simulink model "Controller_Pioneer3DXAssembly"  (R2019b)
settings: Solver=ode45  StartTime=0.0  StopTime=200  RelTol=1e-3  EnableMultiTasking=on
InitFcn:
  | load WorldLUTData.mat
  | r = 0.095; %Wheel radius
  | b = 0.33; %Wheel base
undefined symbols (not defined in the file): World_LUT, X, Y, Z
libraries: sm_lib x35, nesl_utility x19, fl_lib x3, fl_ps_legacy_lib x3, vrlib x2
(part 2 of 2)

== system Controller_Pioneer3DXAssembly/Wheel Right/WheelMain_1_RIGID ==
  ReferenceFrame : sm_lib/Frames and Transforms/Reference Frame
  Solid : sm_lib/Body Elements/File Solid  ExtGeomFileName=WheelMain_Default_sldprt.STL  UnitType=FromFile  ExtGeomFileUnits=in  StepReaderType=HEX  ExportEntireGeometry=off  InertiaType=Custom  Mass=0.95054099999999997  MassUnits=kg  CenterOfMass=[6.6644881889763772 2.3641220472440942e-11 0.063999999999999987]  CenterOfMassUnits=in  MomentsOfInertia=[7.7667865335730646 4.0958211916423819 4.0958211916423819]  MomentsOfInertiaUnits=kg*in^2  ProductsOfInertia=[-2.8456041912083817e-11 2.5874201748403487e-11 1.023105896211792e-11]  ProductsOfInertiaUnits=kg*in^2  BasedOnType=Density  Density=1000  DensityUnits=kg/(m^3)  DoExposeReferenceFrame=on  SerializedFrames=<Frames/>  GraphicType=FromGeometry  MarkerShape=Sphere  MarkerSize=10  MarkerSizeUnits=m  GraphicVisPropType=SimpleVisualProperties  GraphicDiffuseColor=[0.792157 0.819608 0.933333]  GraphicSpecularColor=[0.5 0.5 0.5 1.0]  GraphicAmbientColor=[0.15 0.15 0.15 1.0]  GraphicEmissiveColor=[0.0 0.0 0.0 1.0]  GraphicShininess=75  GraphicOpacity=1
  Transform : sm_lib/Frames and Transforms/Rigid Transform  TranslationMethod=Cartesian  TranslationStandardOffset=0  TranslationLengthUnit=m  TranslationStandardAxis=+Z  TranslationCartesianOffset=[0.18929299999999999 -5.2736824223548195e-08 0.001625527193626478]  TranslationROffset=0  TranslationROffsetUnits=m  TranslationZOffset=0  TranslationZOffsetUnits=m  TranslationThetaOffset=0  TranslationThetaOffsetUnits=deg  RotationMethod=ArbitraryAxis  RotationAngleUnits=rad  RotationStandardAxis=+Z  RotationAngle=2.0943951023931957  RotationArbitraryAxis=[-0.57735026918962584 -0.57735026918962573 0.57735026918962573]  FollAlignAxisA=+X  BaseAlignAxisA=+Y  FollAlignAxisB=+Y  BaseAlignAxisB=+Z  RotationSequenceAxes=FollowerAxes  RotationSequence=XYX  RotationSequenceAngles=[0 0 0]  RotationSequenceAnglesUnits=deg  RotationMatrix=[1 0 0; 0 1 0; 0 0 1]
  F : PMIOPort  Side=Left
  connections:
  Transform/RConn1 -- F/RConn1
  Transform/LConn1 -- ReferenceFrame/RConn1 -- Solid/RConn1

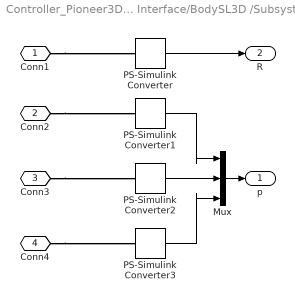
== system Controller_Pioneer3DXAssembly/SM-->SL3D Interface/BodySL3D /Subsystem ==
  Mux : Mux  Inputs=3
  PS-Simulink Converter{,1..3} (4 alike) : nesl_utility/PS-Simulink Converter  PhysicalDomain=network_engine_domain  SubClassName=ps_output  LeftPortType=input  RightPortType=output  PseudoPeriodic=off  Frequencies=[]  Unit=1  AffineConversion=off
  Conn1 : PMIOPort  Side=Left
  Conn2 : PMIOPort  Port=2  Side=Left
  Conn3 : PMIOPort  Port=3  Side=Left
  Conn4 : PMIOPort  Port=4  Side=Left
  p : Outport
  R : Outport  Port=2
  wires:
  PS-Simulink Converter/1 -> R/1
  Mux/1 -> p/1
  PS-Simulink Converter1/1 -> Mux/1
  PS-Simulink Converter2/1 -> Mux/2
  PS-Simulink Converter3/1 -> Mux/3
  connections:
  Conn1/RConn1 -- PS-Simulink Converter/LConn1
  Conn3/RConn1 -- PS-Simulink Converter2/LConn1
  Conn4/RConn1 -- PS-Simulink Converter3/LConn1
  Conn2/RConn1 -- PS-Simulink Converter1/LConn1

== system Controller_Pioneer3DXAssembly/SM-->SL3D Interface/CCSL3D/Subsystem ==
  PS-Simulink Converter : nesl_utility/PS-Simulink Converter  PhysicalDomain=network_engine_domain  SubClassName=ps_output  LeftPortType=input  RightPortType=output  PseudoPeriodic=off  Frequencies=[]  Unit=1  AffineConversion=off
  Conn1 : PMIOPort  Side=Left
  Omega_z : Outport
  wires:
  PS-Simulink Converter/1 -> Omega_z/1
  connections:
  Conn1/RConn1 -- PS-Simulink Converter/LConn1

== system Controller_Pioneer3DXAssembly/SM-->SL3D Interface/CWSL3D/Subsystem ==
  PS-Simulink Converter : nesl_utility/PS-Simulink Converter  PhysicalDomain=network_engine_domain  SubClassName=ps_output  LeftPortType=input  RightPortType=output  PseudoPeriodic=off  Frequencies=[]  Unit=1  AffineConversion=off
  Conn1 : PMIOPort  Side=Left
  Omega_z : Outport
  wires:
  PS-Simulink Converter/1 -> Omega_z/1
  connections:
  Conn1/RConn1 -- PS-Simulink Converter/LConn1

== system Controller_Pioneer3DXAssembly/SM-->SL3D Interface/LWSL3D/Subsystem ==
  PS-Simulink Converter : nesl_utility/PS-Simulink Converter  PhysicalDomain=network_engine_domain  SubClassName=ps_output  LeftPortType=input  RightPortType=output  PseudoPeriodic=off  Frequencies=[]  Unit=1  AffineConversion=off
  Conn1 : PMIOPort  Side=Left
  Omega_z : Outport
  wires:
  PS-Simulink Converter/1 -> Omega_z/1
  connections:
  Conn1/RConn1 -- PS-Simulink Converter/LConn1

== system Controller_Pioneer3DXAssembly/SM-->SL3D Interface/RWSL3D/Subsystem ==
  PS-Simulink Converter : nesl_utility/PS-Simulink Converter  PhysicalDomain=network_engine_domain  SubClassName=ps_output  LeftPortType=input  RightPortType=output  PseudoPeriodic=off  Frequencies=[]  Unit=1  AffineConversion=off
  Conn1 : PMIOPort  Side=Left
  Omega_z : Outport
  wires:
  PS-Simulink Converter/1 -> Omega_z/1
  connections:
  Conn1/RConn1 -- PS-Simulink Converter/LConn1

== stateflow chart Controller_Pioneer3DXAssembly/Control Algorithm ==
  state Modes
    en,du:
    frontSensors = SonarSensors(4:5) < SensorRanges(4:5);
    leftMostSensors = [SonarSensors(1)] < SensorRanges(1);
    leftMiddleSensors = [SonarSensors(2:3)] < SensorRanges(2:3);
    rightMiddleSensors = [SonarSensors(6:7)] < SensorRanges(6:7);
    rightMostSensors = [SonarSensors(8) ]< SensorRanges(8);
    state ReverseABit
      en,du:
      RightVel = -v0;
      LeftVel = -v0;
    state GoStraight
      en,du:
      RightVel = v0;
      LeftVel = v0;
    state DetermineLeftRight
    state TurnRightInPlace
      du :
      RightVel = -v0;
      LeftVel = v0;
    state TurnLeftInPlace
      du :
      RightVel = v0;
      LeftVel = -v0;
    state TurnRightTight
      du :
      RightVel = v0/5;
      LeftVel = v0;
    state TurnLeftTight
      du :
      RightVel = v0;
      LeftVel = v0/5;
    state TurnRightWide
      du:
      RightVel = v0/2;
      LeftVel = v0;
    state TurnLeftWide
      du :
      RightVel = v0;
      LeftVel = v0/2;
    (default) -> ReverseABit
    ReverseABit -> GoStraight : after(3,sec)
    TurnRightWide -> GoStraight : [all(leftMostSensors<1)]
    GoStraight -> TurnRightWide [order 4] : [any(leftMostSensors>0)]
    TurnRightTight -> GoStraight : [all(leftMiddleSensors<1)]
    GoStraight -> TurnRightTight [order 2] : [any(leftMiddleSensors>0)]
    TurnRightInPlace -> GoStraight : [all(frontSensors<1)]
    GoStraight -> DetermineLeftRight [order 1] : [any(frontSensors>0)]
    TurnLeftInPlace -> GoStraight : [all(frontSensors<1)]
    TurnLeftTight -> GoStraight : [all(rightMiddleSensors<1)]
    GoStraight -> TurnLeftTight [order 3] : [any(rightMiddleSensors>0)]
    TurnLeftWide -> GoStraight : [all(rightMostSensors<1)]
    GoStraight -> TurnLeftWide [order 5] : [any(rightMostSensors>0)]
    DetermineLeftRight -> TurnRightInPlace [order 1] : [SonarSensors(4)>SonarSensors(5)]
    DetermineLeftRight -> TurnLeftInPlace [order 2] : %default
  data: LeftVel output; RightVel output; SonarSensors input; frontSensors local; SensorRanges input; v0 parameter; leftMostSensors local; leftMiddleSensors local; rightMostSensors local; rightMiddleSensors local

== matlab function Controller_Pioneer3DXAssembly/Virtual Sensors Subsystem/MATLAB Function ==
  data: x input; y input; rotMat input; xRange output; yRange output; r_range parameter size=8
function [xRange, yRange] = getVirtualBox(x,y,rotMat, r_range)
%#codegen
%% Dimensions
r_com = 0.27/2;%Radius of the SONAR arc in 'm'
r_range_m = r_range/1000;
% r_range = 0.5;%Radius of SONAR range in 'm'
r_b = r_com + r_range_m;%Back SONAR arc radius
yb_b = 0.18;%Shift in Y axis from COM

r_f = r_com + r_range_m;%Front SONAR arc radius, same as back in our case
yb_f = 0.09;%Shift in Y axis from COM

SensorPos = zeros(16,2);
SensorPosNew = zeros(16,3);
%% FRONT SENSORS
SensorPos(1,:) = [r_f(1)*sind(-90), r_f(1)*cosd(-90)+yb_f];
SensorPos(8,:) = [r_f(8)*sind(90), r_f(8)*cosd(90)+yb_f];

%Remaining front sensors
i = 2;
for theta = -50:20:50
    SensorPos(i,:) = [r_f(i)*sind(theta), r_f(i)*cosd(theta)+yb_f];
    i = i+1;
end

%% BACK SENSORS
SensorPos(9,:) = [r_b(1)*sind(90), r_b(1)*cosd(90)-yb_b];
SensorPos(16,:) = [r_b(8)*sind(-90), r_b(8)*cosd(-90)-yb_b];

%Remaining back sensors
i = 10;
for theta = -50:20:50
    SensorPos(i,:) = [-r_b(i-8)*sind(theta), -r_b(i-8)*cosd(theta)-yb_b];
    i = i+1;
end
rotZ90 = [0 -1 0; 1 0 0; 0 0 1];
rotMatNew = rotMat * rotZ90;
for i = 1:16
    SensorPosNew(i,:) = (rotMatNew*[SensorPos(i,:)';0] + [x; y;0])';
end

xRange = SensorPosNew(:,1);%Inp(:,1);
yRange = SensorPosNew(:,2);%-Inp(:,2);
